simulink model "PD_FLC_simulink"  (R2018a)
settings: Solver=FixedStepAuto  StartTime=0.0  StopTime=t_end  FixedStep=0.001  MaxStep=0.01  MinStep=1e-4  RelTol=1e-3
values from neighbouring files (symbols this model uses):
  Den = [1 12 24]    [GA_Ks.m]
  K = bestK    (= 0)    [GA_Ks.m]
  Kd = bestKd    (= 0)    [GA_Ks.m]
  Kp = bestKp    (= 0)    [GA_Ks.m]
  Num = [2]    [GA_Ks.m]
libraries: fuzblock x1
settings Model: SimulationMode=accelerator  Creator=Milosh Yokich  LastModifiedBy=Milosh Yokich

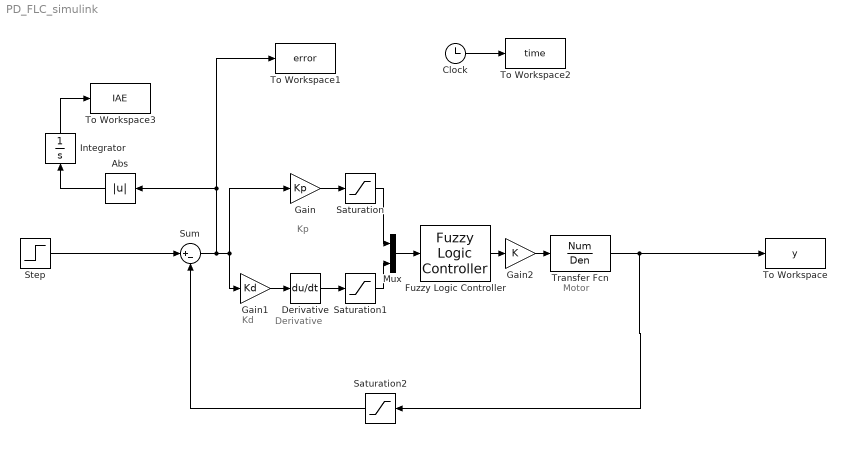
== system PD_FLC_simulink ==
  note: Derivative
  note: Motor
  note: Kd
  note: Kp
  Abs : Abs
  Clock : Clock
  Derivative : Derivative  CoefficientInTFapproximation=0.000000000001
  Fuzzy Logic Controller : fuzblock/Fuzzy Logic  Controller  FIS=fis  OutputSampleNumber=101  DataType=double  FuzzifiedInputs=off  RuleFiringStrengths=off  RuleOutputs=off  AggregatedOutputs=off  SimulateUsing=Code generation  OutOfRangeInputValueMessage=none  NoRuleFiredMessage=none  EmptyOutputFuzzySetMessage=none
  Gain : Gain  Gain=Kp
  Gain1 : Gain  Gain=Kd
  Gain2 : Gain  Gain=K
  Integrator : Integrator
  Mux : Mux  Inputs=2
  Saturation : Saturate  UpperLimit=1  LowerLimit=-1
  Saturation1 : Saturate  UpperLimit=1  LowerLimit=-1
  Saturation2 : Saturate  UpperLimit=10  LowerLimit=-10
  Step : Step  Time=0.01  SampleTime=0
  Sum : Sum  Inputs=|+-
  To Workspace : ToWorkspace  VariableName=y  SampleTime=-1
  To Workspace1 : ToWorkspace  VariableName=error  SampleTime=-1
  To Workspace2 : ToWorkspace  VariableName=time  SampleTime=-1
  To Workspace3 : ToWorkspace  VariableName=IAE  SampleTime=-1
  Transfer Fcn : TransferFcn  Numerator=Num  Denominator=Den
  wires:
  Step/1 -> Sum/1
  Sum/1 -> Gain/1, Gain1/1, To Workspace1/1, Abs/1
  Gain1/1 -> Derivative/1
  Clock/1 -> To Workspace2/1
  Transfer Fcn/1 -> To Workspace/1, Saturation2/1
  Fuzzy Logic Controller/1 -> Gain2/1
  Gain2/1 -> Transfer Fcn/1
  Mux/1 -> Fuzzy Logic Controller/1
  Derivative/1 -> Saturation1/1
  Gain/1 -> Saturation/1
  Saturation/1 -> Mux/1
  Saturation1/1 -> Mux/2
  Abs/1 -> Integrator/1
  Integrator/1 -> To Workspace3/1
  Saturation2/1 -> Sum/2
